simulink model "Problem_2"  (R2020a)
settings: Solver=VariableStepAuto  StartTime=0.0  StopTime=30  RelTol=1e-3
PreLoadFcn:
  | m1 = 2500;
  | m2 = 320;
  | k1 = 80000;
  | k2 = 500000;
  | b = 350;
undefined symbols (not defined in the file): sigbuilder_block
settings Model: Creator=Ganesh  LastModifiedBy=Ganesh

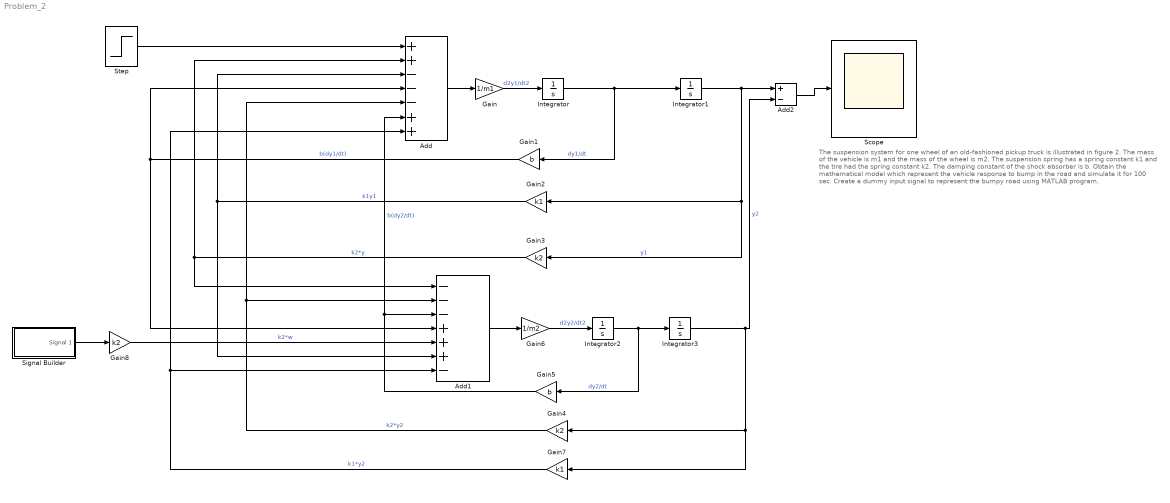
== system Problem_2 ==
  note: The suspension system for one wheel of an old-fashioned pickup truck is illustrated in figure 2. The mass of the vehicle is m1 and the mass of the wheel is m2. The suspension spring has a spring constant k1 and the tire had the spring constant k2. The damping constant of the shock absorber is b. Obtain the mathematical model which represent the vehicle response to bump in the road and simulate it for 100 sec. Create a dummy input signal to represent the bumpy road using MATLAB program.
  Add : Sum  Inputs=++---++
  Add1 : Sum  Inputs=---+++-
  Add2 : Sum  Inputs=+-
  Gain : Gain  Gain=1/m1
  Gain1 : Gain  Gain=b
  Gain2 : Gain  Gain=k1
  Gain3 : Gain  Gain=k2
  Gain4 : Gain  Gain=k2
  Gain5 : Gain  Gain=b
  Gain6 : Gain  Gain=1/m2
  Gain7 : Gain  Gain=k1
  Gain8 : Gain  Gain=k2
  Integrator{,1..3} (4 alike) : Integrator
  Scope : Scope
  Signal Builder : Subsystem  Tag=STV Subsys  LoadFcn=sigbuilder_block('load');  StartFcn=sigbuilder_block('start');  StopFcn=sigbuilder_block('stop');  ClipboardFcn=sigbuilder_block('clipboard');  mask(Sigbuilder block){tuvar=[0:10]}
      mask help: Simulink:masks:SigbuilderBlock_MD
      mask init:
      | if ~strcmp(get_param(bdroot(gcbh),'SimulationStatus'),'stopped') tuvar = sigbuilder_block('maskInit'); end
      settings: CopyFcn=sigbuilder_block('copy');  DeleteFcn=sigbuilder_block('delete');  ModelCloseFcn=sigbuilder_block('modelClose');  PreSaveFcn=sigbuilder_block('preSave');  PauseFcn=sigbuilder_block('pause');  ContinueFcn=sigbuilder_block('continue');  NameChangeFcn=sigbuilder_block('namechange');  OpenFcn=sigbuilder_block('open',[424.2 130.2 550.8 400.2 ]);  CloseFcn=sigbuilder_block('close');
      mask Display: plot(0, 0, 100, 100,[2, 2, 32, 32, 2], [68, 8, 8, 68, 68],[32, 2], [38, 38], [32, 19, 2],[53, 60, 44], [32, 17, 17, 2],[16, 16, 31, 31]);txt = getActiveGroup(gcbh);text(2, 100, txt,'verticalAlignment', 'top');
  Step : Step  SampleTime=0
  wires:
  Add/1 -> Gain/1
  Gain/1 -> Integrator/1  "d2y1/dt2"
  Integrator/1 -> Integrator1/1, Gain1/1  "dy1/dt"
  Integrator1/1 -> Add2/1, Gain2/1, Gain3/1  "y1"
  Gain1/1 -> Add/4, Add1/4  "b(dy1/dt)"
  Gain3/1 -> Add/2, Add1/1  "k2*y"
  Add1/1 -> Gain6/1
  Gain6/1 -> Integrator2/1  "d2y2/dt2"
  Integrator2/1 -> Integrator3/1, Gain5/1  "dy2/dt"
  Integrator3/1 -> Gain7/1, Gain4/1, Add2/2  "y2"
  Gain4/1 -> Add/5, Add1/2  "k2*y2"
  Gain5/1 -> Add1/3, Add/6  "b(dy2/dt)"
  Gain7/1 -> Add/7, Add1/7  "k1*y2"
  Signal Builder/1(Signal 1) -> Gain8/1
  Gain2/1 -> Add1/6, Add/3  "k1y1"
  Gain8/1 -> Add1/5  "k2*w"
  Add2/1 -> Scope/1
  Step/1 -> Add/1

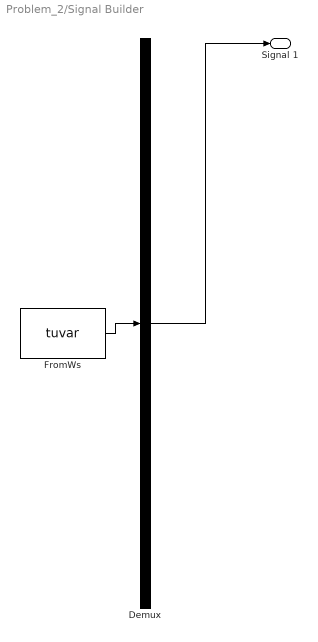
== system Problem_2/Signal Builder ==
  Demux : Demux  Tag=STV Demux  Outputs=1
      settings: DisplayOption=none
  FromWs : FromWorkspace  Tag=STV FromWs  VariableName=tuvar
      SigBuilderData=|
      | common.afterFinalStr = 'Extrapolate'
      | common.sampleTime = 0
      | dataSet.timeRange = [0 10]
      | dataSet.name = 'Group 1'
      | sbobj.Groups.Name = 'Group 1'
      | sbobj.Groups.Signals.Name = 'Signal 1'
      | sbobj.Groups.Signals.XData = [0 4 4 6 6 10]
      | sbobj.Groups.Signals.YData = [-0.005 0.425 0.765 0.79 0.465 0]
  Signal 1 : Outport  Tag=STV Outport
  wires:
  Demux/1 -> Signal 1/1
  FromWs/1 -> Demux/1
